simulink model "sampleModel1572_3_sub_sub"  (R2023a)
settings: Solver=VariableStepAuto  StartTime=0.0  StopTime=10.0  RelTol=1e-3
libraries: hdlsllib x3, simulink x1
settings Model: Creator=user1  LastModifiedBy=user1

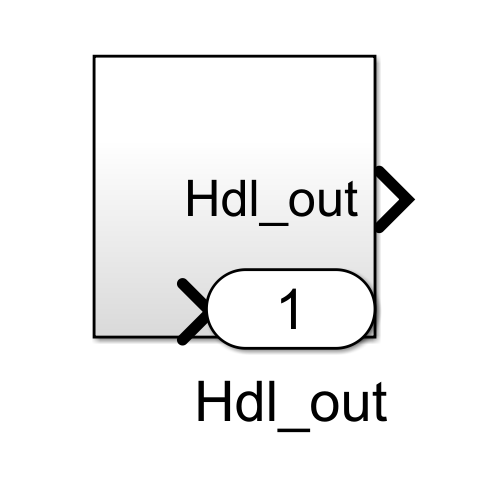
[thumbnail: Simulink's stored preview of the top-level diagram]
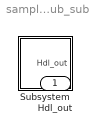
== system sampleModel1572_3_sub_sub ==
  Subsystem : Subsystem
  Hdl_out : Outport  OutDataTypeStr=uint8

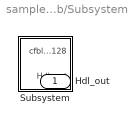
== system sampleModel1572_3_sub_sub/Subsystem ==
  Subsystem : Subsystem
  Hdl_out : Outport  OutDataTypeStr=uint8

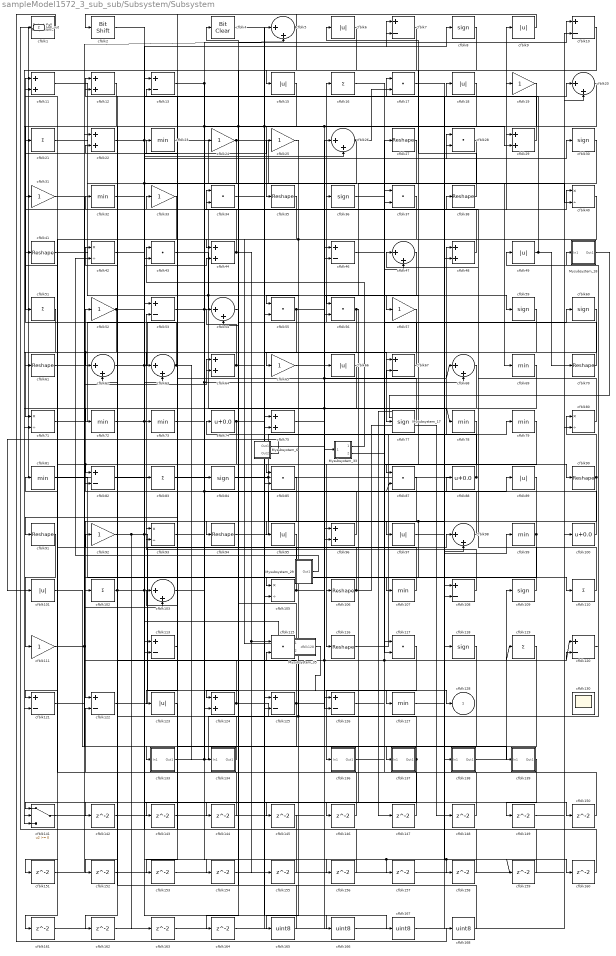
== system sampleModel1572_3_sub_sub/Subsystem/Subsystem ==
  Mysubsystem_17 : Subsystem  TreatAsAtomicUnit=on  RTWFcnName=Mysubsystem_17
      settings: RTWFcnNameOpts=User specified  RTWFileNameOpts=Use function name
  Mysubsystem_18 : Subsystem  TreatAsAtomicUnit=on  RTWFcnName=Mysubsystem_18
      settings: RTWFcnNameOpts=User specified  RTWFileNameOpts=Use function name
  Mysubsystem_29 : Subsystem  TreatAsAtomicUnit=on  RTWFcnName=Mysubsystem_29
      settings: RTWFcnNameOpts=User specified  RTWFileNameOpts=Use function name
  Mysubsystem_33 : Subsystem  TreatAsAtomicUnit=on  RTWFcnName=Mysubsystem_33
      settings: RTWFcnNameOpts=User specified  RTWFileNameOpts=Use function name
  Mysubsystem_35 : Subsystem  TreatAsAtomicUnit=on  RTWFcnName=Mysubsystem_35
      settings: RTWFcnNameOpts=User specified  RTWFileNameOpts=Use function name
  Mysubsystem_6 : Subsystem  TreatAsAtomicUnit=on  RTWFcnName=Mysubsystem_6
      settings: RTWFcnNameOpts=User specified  RTWFileNameOpts=Use function name
  cfblk1 : hdlsllib/Logic and Bit Operations/Detect Fall Nonpositive  vinit=0  OutDataTypeStr=uint8
  cfblk{7,10,13,46,53,67,82,108,113,120..122,125..126} (14 alike) : Sum  Inputs=+-  OutDataTypeStr=uint8
  cfblk100 : Bias  Bias=0.0  SaturateOnIntegerOverflow=off
  cfblk{6,9,15,18,49,66,89,95,97,101,123} (11 alike) : Abs  OutDataTypeStr=uint8  SaturateOnIntegerOverflow=off
  cfblk{16,21,51,83,102,110,119} (7 alike) : Sum  Inputs=+  OutDataTypeStr=uint8
  cfblk{5,20,26,47,54,62..63,68,98,103} (10 alike) : Sum  Inputs=|++  OutDataTypeStr=uint8
  cfblk{40,42,71,80,93,105} (6 alike) : Product  Inputs=*/  OutDataTypeStr=uint8  RndMeth=Zero  SaturateOnIntegerOverflow=on
  cfblk{27,35,38,41,61,70,90..91,94,106,116} (11 alike) : Reshape
  cfblk{23,32,69,72..73,78..79,81,99,107,127} (11 alike) : MinMax  OutDataTypeStr=uint8
  cfblk{8,30,36,59..60,77,84,109,118} (9 alike) : Signum
  cfblk{11..12,22,29,44,48,64,75,96,124} (10 alike) : Sum  OutDataTypeStr=uint8
  cfblk{19,24..25,31,33,52,57,65,92,111} (10 alike) : Gain  OutDataTypeStr=uint8
  cfblk{17,28,34,37,43,55..56,85,87,115,117} (11 alike) : DotProduct  OutDataTypeStr=uint8
  cfblk130 : Scope
      settings: Floating=on
  cfblk133 : Subsystem
      settings: LibrarySourceBlock=|
      | hdlsllib/Ports &
      | Subsystems/Subsystem
  cfblk134 : Subsystem
      settings: LibrarySourceBlock=|
      | hdlsllib/Ports &
      | Subsystems/Subsystem
  cfblk136 : Subsystem
      settings: LibrarySourceBlock=|
      | hdlsllib/Ports &
      | Subsystems/Subsystem
  cfblk137 : Subsystem
      settings: LibrarySourceBlock=|
      | hdlsllib/Ports &
      | Subsystems/Subsystem
  cfblk138 : Subsystem
      settings: LibrarySourceBlock=|
      | hdlsllib/Ports &
      | Subsystems/Subsystem
  cfblk139 : Subsystem
      settings: LibrarySourceBlock=|
      | hdlsllib/Ports &
      | Subsystems/Subsystem
  cfblk141 : Switch  OutDataTypeStr=uint8  SaturateOnIntegerOverflow=off  InputSameDT=off
  cfblk{142..164} (23 alike) : Delay  SampleTime=1
  cfblk{165..168} (4 alike) : DataTypeConversion  OutDataTypeStr=uint8  SaturateOnIntegerOverflow=off  RndMeth=Floor
  cfblk2 : hdlsllib/Logic and Bit Operations/Bit Shift  mode=Shift Left Logical  N=0
  cfblk4 : simulink/Logic and Bit Operations/Bit Clear  iBit=0
      settings: LibrarySourceBlock=|
      | hdlsllib/Logic and Bit
      | Operations/Bit Clear
  cfblk74 : Bias  Bias=0.0  SaturateOnIntegerOverflow=off
  cfblk88 : Bias  Bias=0.0  SaturateOnIntegerOverflow=off
  cfblk128 : Outport  OutDataTypeStr=uint8  VectorParamsAs1DForOutWhenUnconnected=off
  Hdl_out : Outport  Port=2  OutDataTypeStr=uint8
  wires:
  Mysubsystem_35/1(cfblk128) -> cfblk128/1
  cfblk40/1 -> Mysubsystem_35/1(In1)
  Mysubsystem_33/2(Out2) -> cfblk117/1
  Mysubsystem_33/1(Out1) -> cfblk43/1
  Mysubsystem_6/1(Out1) -> Mysubsystem_33/1(In1)
  Mysubsystem_29/1(Out1) -> cfblk42/2
  Mysubsystem_18/1(Out1) -> Mysubsystem_17/1(In1)
  cfblk120/1 -> Mysubsystem_18/1(In1)
  Mysubsystem_17/2(Out2) -> cfblk148/1
  Mysubsystem_17/1(Out1) -> cfblk147/1
  Mysubsystem_6/2(Out2) -> cfblk101/1
  cfblk168/1 -> cfblk32/1
  cfblk1/1 -> cfblk168/1
  cfblk167/1 -> cfblk100/1
  cfblk32/1 -> cfblk167/1
  cfblk166/1 -> cfblk48/2
  cfblk4/1 -> cfblk166/1
  cfblk165/1 -> cfblk4/1
  cfblk57/1 -> cfblk165/1
  cfblk164/1 -> cfblk108/2
  cfblk163/1 -> cfblk125/1
  cfblk162/1 -> cfblk46/2
  cfblk161/1 -> cfblk26/1
  cfblk160/1 -> cfblk53/1
  cfblk17/1 -> cfblk160/1
  cfblk159/1 -> cfblk93/2
  cfblk158/1 -> cfblk13/1
  cfblk157/1 -> cfblk20/2
  cfblk156/1 -> cfblk62/2
  cfblk155/1 -> cfblk113/1
  cfblk154/1 -> cfblk96/1
  cfblk153/1 -> cfblk10/2
  cfblk118/1 -> cfblk153/1
  cfblk152/1 -> cfblk5/1
  cfblk151/1 -> cfblk22/1
  cfblk33/1 -> cfblk151/1
  cfblk150/1 -> cfblk122/2
  cfblk149/1 -> cfblk80/2
  cfblk139/1(Out1) -> cfblk149/1
  cfblk148/1 -> cfblk37/1
  cfblk147/1 -> cfblk64/2
  cfblk146/1 -> cfblk126/1
  cfblk69/1 -> cfblk146/1
  cfblk145/1 -> cfblk1/1
  cfblk73/1 -> cfblk145/1
  cfblk144/1 -> cfblk11/2
  cfblk54/1 -> cfblk144/1
  cfblk143/1 -> cfblk75/1
  cfblk123/1 -> cfblk143/1
  cfblk142/1 -> cfblk63/2
  cfblk47/1 -> cfblk126/2
  cfblk12/1 -> cfblk71/2
  cfblk83/1 -> cfblk7/1
  cfblk102/1 -> Mysubsystem_35/2(In2), cfblk28/1, cfblk142/1
  cfblk77/1 -> cfblk21/1
  cfblk30/1 -> cfblk87/1
  cfblk68/1 -> cfblk121/2
  cfblk35/1 -> cfblk121/1
  cfblk127/1 -> cfblk99/1
  cfblk26/1 -> cfblk63/1, cfblk17/2
  cfblk51/1 -> cfblk71/1
  cfblk113/1 -> cfblk93/1
  cfblk107/1 -> cfblk12/2
  cfblk24/1 -> cfblk113/2, cfblk40/2
  cfblk70/1 -> cfblk31/1
  cfblk34/1 -> cfblk30/1
  cfblk8/1 -> cfblk57/1
  cfblk89/1 -> cfblk82/2
  cfblk27/1 -> cfblk56/1
  cfblk106/1 -> Mysubsystem_17/2(In2), cfblk41/1
  cfblk49/1 -> cfblk19/1, cfblk70/1
  cfblk2/1 -> cfblk26/2
  cfblk125/1 -> cfblk119/1, cfblk67/2, cfblk83/1, cfblk164/1
  cfblk61/1 -> cfblk103/2
  cfblk81/1 -> cfblk124/2
  cfblk21/1 -> cfblk73/1, cfblk69/1
  cfblk100/1 -> cfblk23/1
  cfblk121/1 -> cfblk64/1
  cfblk44/1 -> cfblk115/1, cfblk155/1, cfblk13/2
  cfblk13/1 -> cfblk29/2, cfblk156/1, cfblk7/2
  cfblk36/1 -> cfblk27/1
  cfblk18/1 -> cfblk51/1
  cfblk84/1 -> cfblk79/1, cfblk118/1
  cfblk55/1 -> cfblk102/1, cfblk59/1
  cfblk134/1(Out1) -> cfblk103/1
  cfblk110/1 -> cfblk88/1
  cfblk136/1(Out1) -> cfblk40/1
  cfblk65/1 -> cfblk97/1
  cfblk93/1 -> cfblk38/1
  cfblk137/1(Out1) -> cfblk92/1, cfblk115/2, cfblk161/1
  cfblk37/1 -> cfblk123/1, cfblk85/1
  cfblk115/1 -> cfblk54/2
  cfblk10/1 -> cfblk55/2
  cfblk25/1 -> cfblk55/1
  cfblk46/1 -> cfblk90/1
  cfblk22/1 -> cfblk8/1, cfblk150/1
  cfblk16/1 -> cfblk47/2
  cfblk19/1 -> cfblk35/1
  cfblk82/1 -> cfblk158/1, cfblk159/1, cfblk157/1
  cfblk103/1 -> cfblk24/1
  cfblk5/1 -> cfblk2/1, cfblk141/2
  cfblk66/1 -> cfblk95/1
  cfblk111/1 -> cfblk5/2, cfblk120/2
  cfblk28/1 -> cfblk37/2
  cfblk105/1 -> cfblk81/1, cfblk29/1
  cfblk31/1 -> cfblk139/1(In1)
  cfblk133/1(Out1) -> cfblk28/2, cfblk68/2, cfblk87/2, cfblk98/2
  cfblk56/1 -> cfblk106/1, cfblk61/1
  cfblk78/1 -> cfblk82/1, cfblk141/1
  cfblk75/1 -> cfblk46/1, cfblk68/1, cfblk78/1
  cfblk91/1 -> cfblk111/1
  cfblk90/1 -> cfblk125/2, cfblk107/1, cfblk80/1
  cfblk108/1 -> cfblk53/2
  cfblk23/1 -> cfblk108/1
  cfblk20/1 -> cfblk124/1, cfblk85/2, cfblk96/2
  cfblk96/1 -> cfblk42/1
  cfblk62/1 -> cfblk10/1, cfblk25/1
  cfblk42/1 -> cfblk110/1
  cfblk94/1 -> cfblk89/1
  cfblk85/1 -> cfblk105/2
  cfblk7/1 -> cfblk94/1
  cfblk52/1 -> cfblk62/1, cfblk141/3, cfblk17/1
  cfblk15/1 -> cfblk72/1, cfblk44/1
  cfblk116/1 -> cfblk48/1
  cfblk41/1 -> cfblk84/1
  cfblk119/1 -> cfblk137/1(In1)
  cfblk64/1 -> cfblk54/1, cfblk67/1
  cfblk6/1 -> cfblk15/1
  cfblk11/1 -> cfblk75/2
  cfblk29/1 -> cfblk12/1
  cfblk126/1 -> cfblk60/1, cfblk120/1
  cfblk71/1 -> cfblk43/2
  cfblk72/1 -> cfblk44/2, cfblk154/1
  cfblk53/1 -> cfblk9/1, cfblk56/2
  cfblk97/1 -> cfblk20/1
  cfblk141/1 -> cfblk66/1
  cfblk43/1 -> cfblk138/1(In1), cfblk117/2
  cfblk79/1 -> cfblk116/1
  cfblk59/1 -> cfblk65/1
  cfblk122/1 -> cfblk98/1
  cfblk38/1 -> cfblk6/1
  cfblk109/1 -> cfblk47/1
  cfblk98/1 -> cfblk52/1
  cfblk60/1 -> cfblk77/1
  cfblk95/1 -> cfblk105/1
  cfblk138/1(Out1) -> cfblk109/1
  cfblk117/1 -> cfblk136/1(In1)
  cfblk101/1 -> cfblk133/1(In1)
  cfblk124/1 -> cfblk49/1, cfblk22/2
  cfblk80/1 -> cfblk34/2
  cfblk99/1 -> cfblk34/1, cfblk162/1
  cfblk48/1 -> cfblk33/1
  cfblk9/1 -> cfblk91/1
  cfblk74/1 -> cfblk36/1, cfblk152/1
  cfblk88/1 -> cfblk74/1, Hdl_out/1
  cfblk87/1 -> cfblk122/1
  cfblk63/1 -> cfblk11/1, cfblk134/1(In1)
  cfblk67/1 -> cfblk16/1
  cfblk92/1 -> cfblk127/1, cfblk18/1, cfblk163/1

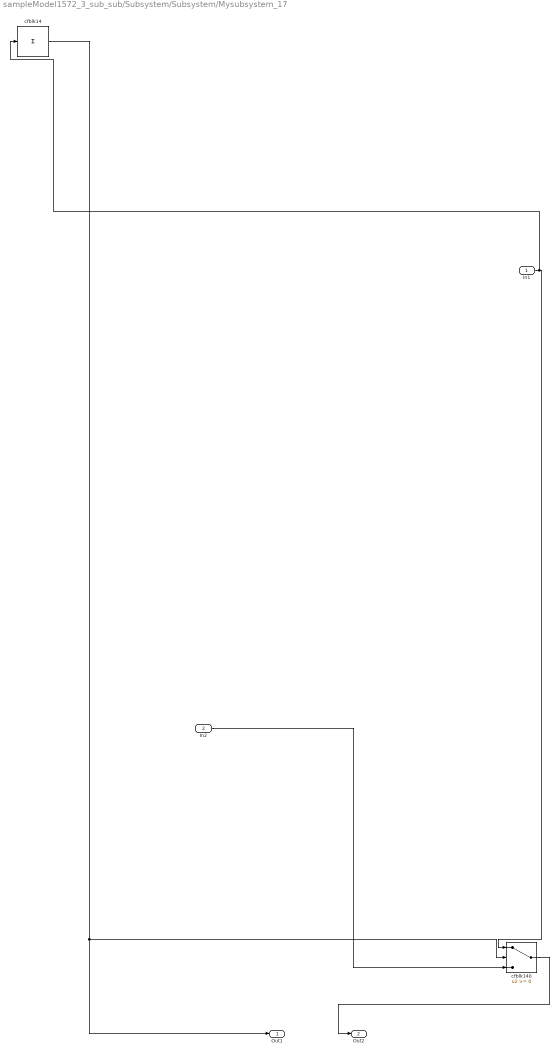
== system sampleModel1572_3_sub_sub/Subsystem/Subsystem/Mysubsystem_17 ==
  In1 : Inport
  In2 : Inport  Port=2
  cfblk14 : Sum  Inputs=+
  cfblk140 : Switch  SaturateOnIntegerOverflow=off  InputSameDT=off
  Out1 : Outport
  Out2 : Outport  Port=2
  wires:
  cfblk14/1 -> Out1/1, cfblk140/2
  cfblk140/1 -> Out2/1
  In1/1 -> cfblk14/1, cfblk140/1
  In2/1 -> cfblk140/3

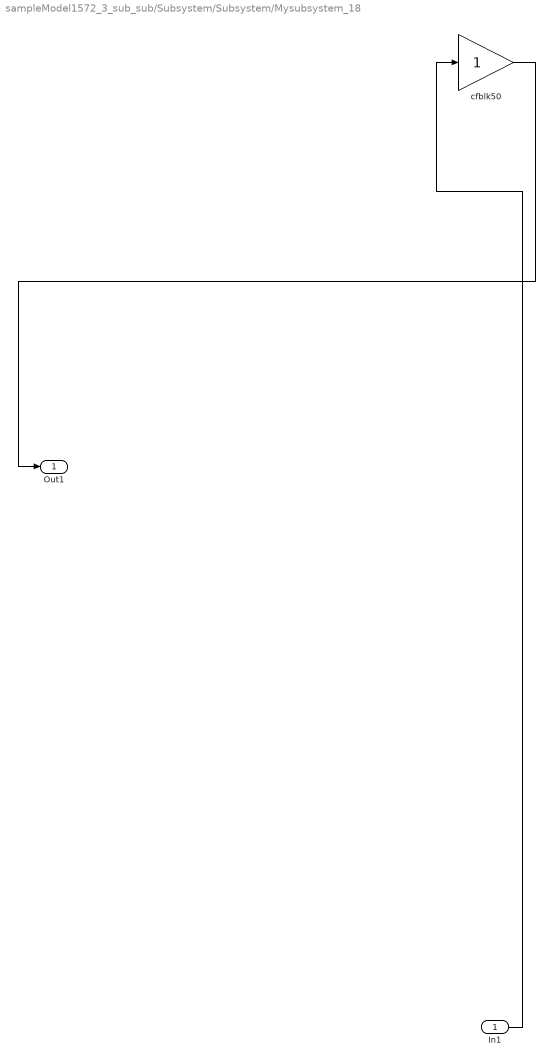
== system sampleModel1572_3_sub_sub/Subsystem/Subsystem/Mysubsystem_18 ==
  In1 : Inport
  cfblk50 : Gain
  Out1 : Outport
  wires:
  cfblk50/1 -> Out1/1
  In1/1 -> cfblk50/1

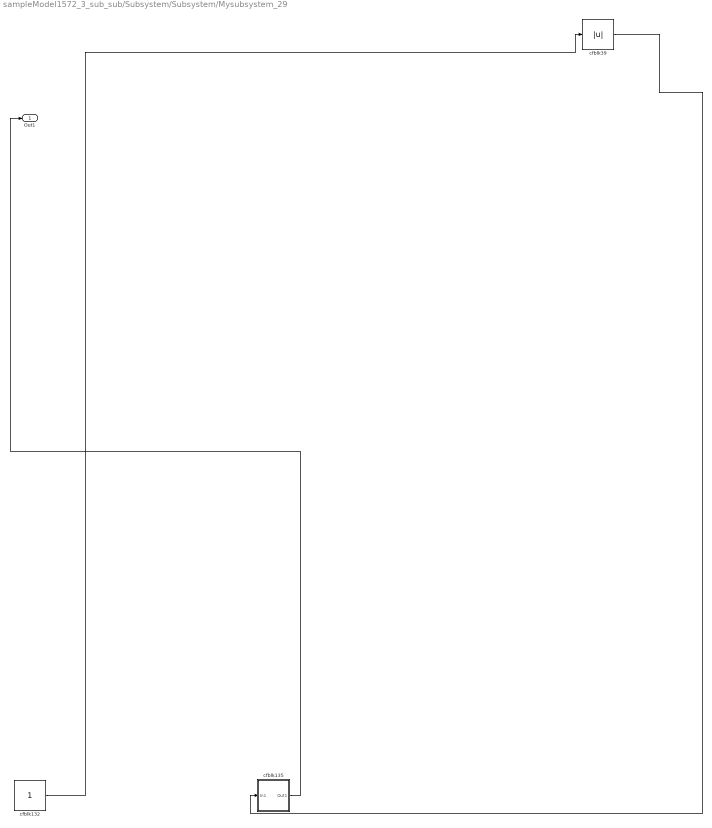
== system sampleModel1572_3_sub_sub/Subsystem/Subsystem/Mysubsystem_29 ==
  cfblk132 : Constant  SampleTime=-1
  cfblk135 : Subsystem
      settings: LibrarySourceBlock=|
      | hdlsllib/Ports &
      | Subsystems/Subsystem
  cfblk39 : Abs  SaturateOnIntegerOverflow=off
  Out1 : Outport
  wires:
  cfblk132/1 -> cfblk39/1
  cfblk135/1(Out1) -> Out1/1
  cfblk39/1 -> cfblk135/1(In1)

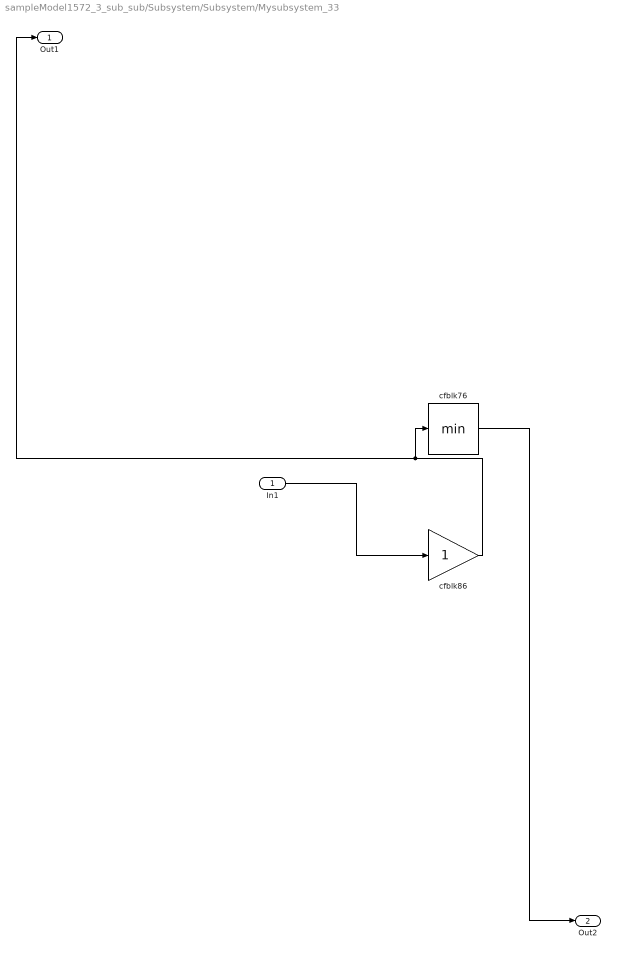
== system sampleModel1572_3_sub_sub/Subsystem/Subsystem/Mysubsystem_33 ==
  In1 : Inport
  cfblk76 : MinMax
  cfblk86 : Gain
  Out1 : Outport
  Out2 : Outport  Port=2
  wires:
  cfblk76/1 -> Out2/1
  cfblk86/1 -> Out1/1, cfblk76/1
  In1/1 -> cfblk86/1

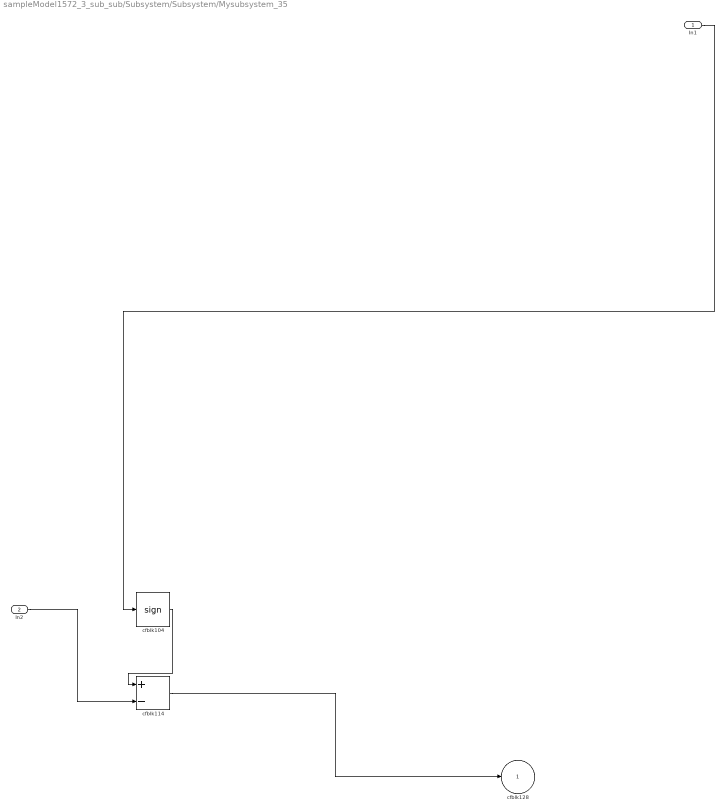
== system sampleModel1572_3_sub_sub/Subsystem/Subsystem/Mysubsystem_35 ==
  In1 : Inport
  In2 : Inport  Port=2
  cfblk104 : Signum
  cfblk114 : Sum  Inputs=+-
  cfblk128 : Outport  VectorParamsAs1DForOutWhenUnconnected=off
  wires:
  cfblk104/1 -> cfblk114/1
  cfblk114/1 -> cfblk128/1
  In1/1 -> cfblk104/1
  In2/1 -> cfblk114/2

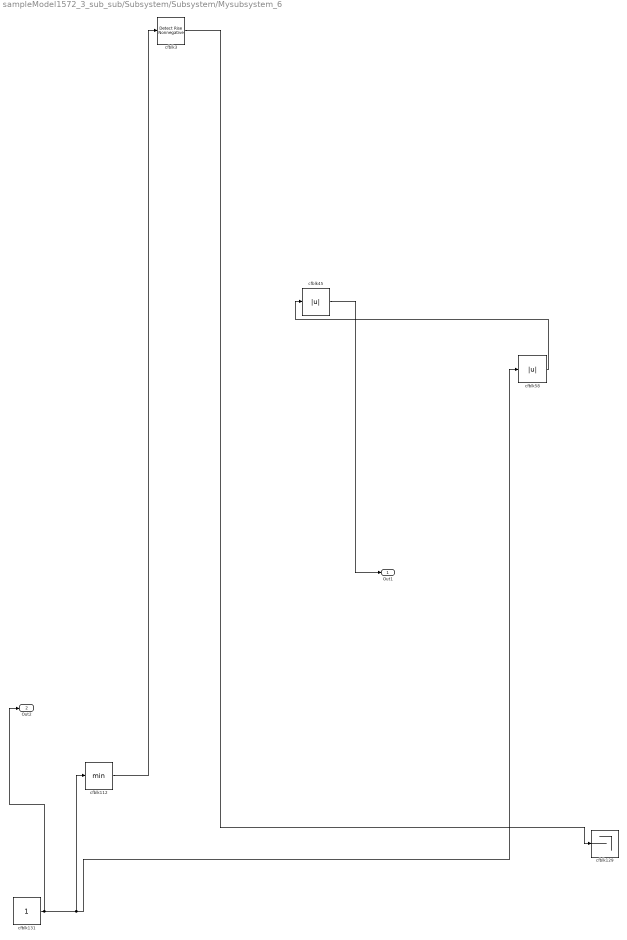
== system sampleModel1572_3_sub_sub/Subsystem/Subsystem/Mysubsystem_6 ==
  cfblk112 : MinMax
  cfblk129 : Terminator
  cfblk131 : Constant  SampleTime=-1
  cfblk3 : hdlsllib/Logic and Bit Operations/Detect Rise Nonnegative  vinit=0  OutDataTypeStr=boolean
  cfblk45 : Abs  SaturateOnIntegerOverflow=off
  cfblk58 : Abs  SaturateOnIntegerOverflow=off
  Out1 : Outport
  Out2 : Outport  Port=2
  wires:
  cfblk3/1 -> cfblk129/1
  cfblk58/1 -> cfblk45/1
  cfblk131/1 -> Out2/1, cfblk112/1, cfblk58/1
  cfblk112/1 -> cfblk3/1
  cfblk45/1 -> Out1/1

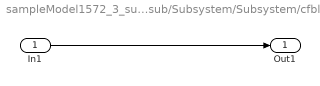
== system sampleModel1572_3_sub_sub/Subsystem/Subsystem/cfblk133 ==
  In1 : Inport
  Out1 : Outport
  wires:
  In1/1 -> Out1/1

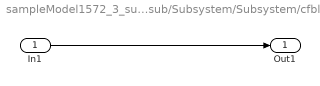
== system sampleModel1572_3_sub_sub/Subsystem/Subsystem/cfblk134 ==
  In1 : Inport
  Out1 : Outport
  wires:
  In1/1 -> Out1/1

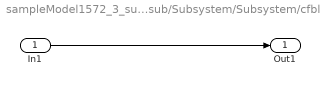
== system sampleModel1572_3_sub_sub/Subsystem/Subsystem/cfblk136 ==
  In1 : Inport
  Out1 : Outport
  wires:
  In1/1 -> Out1/1

== system sampleModel1572_3_sub_sub/Subsystem/Subsystem/cfblk137 ==
  In1 : Inport
  Out1 : Outport
  wires:
  In1/1 -> Out1/1

== system sampleModel1572_3_sub_sub/Subsystem/Subsystem/cfblk138 ==
  In1 : Inport
  Out1 : Outport
  wires:
  In1/1 -> Out1/1

== system sampleModel1572_3_sub_sub/Subsystem/Subsystem/cfblk139 ==
  In1 : Inport
  Out1 : Outport
  wires:
  In1/1 -> Out1/1

== system sampleModel1572_3_sub_sub/Subsystem/Subsystem/Mysubsystem_29/cfblk135 ==
  In1 : Inport
  Out1 : Outport
  wires:
  In1/1 -> Out1/1
